simulink model "EulerKinematicalEquations"  (R2021a)
settings: Solver=FixedStepAuto  StartTime=0.0  StopTime=100  FixedStep=.05  RelTol=1e-3
values from neighbouring files (symbols this model uses):
  Cbv0 = Cb2*C21*C1v    [InitializeModel.m]
  phi0 = 0    [InitializeModel.m]
  psi0 = 0    [InitializeModel.m]
  theta0 = 0.0059    [InitializeModel.m]
settings Model: Creator=Christopher  LastModifiedBy=chris
settings SolverCC: AlgebraicLoopSolver=TrustRegion
settings DataIOCC: ReturnWorkspaceOutputs=off
settings DebuggingCC: SFMachineParentedDataDiag=warning  ArithmeticOperatorsInVariantConditions=warning
settings SFSimCC: CustomCodeUndefinedFunction=UseInterfaceOnly

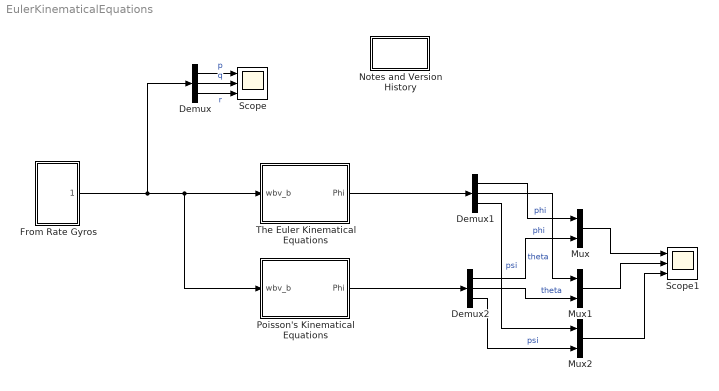
== system EulerKinematicalEquations ==
  Demux : Demux  Outputs=3
  Demux1 : Demux  Outputs=3
  Demux2 : Demux  Outputs=3
  From Rate Gyros : Subsystem
  Mux : Mux  Inputs=2
  Mux1 : Mux  Inputs=2
  Mux2 : Mux  Inputs=2
  Notes and Version History : Subsystem
  Poisson's Kinematical Equations : Subsystem
  Scope : Scope  NumInputPorts=3
  Scope1 : Scope  NumInputPorts=3
  The Euler Kinematical Equations : Subsystem
  wires:
  From Rate Gyros/1(wbv_b) -> Poisson's Kinematical Equations/1(wbv_b), The Euler Kinematical Equations/1(wbv_b), Demux/1
  Demux/1 -> Scope/1  "p"
  Demux/2 -> Scope/2  "q"
  Demux/3 -> Scope/3  "r"
  Demux1/3 -> Mux2/1  "psi"
  Demux1/2 -> Mux1/1  "theta"
  Demux1/1 -> Mux/1  "phi"
  The Euler Kinematical Equations/1(Phi) -> Demux1/1
  Poisson's Kinematical Equations/1(Phi) -> Demux2/1
  Demux2/1 -> Mux/2  "phi"
  Mux/1 -> Scope1/1
  Demux2/2 -> Mux1/2  "theta"
  Mux1/1 -> Scope1/2
  Demux2/3 -> Mux2/2  "psi"
  Mux2/1 -> Scope1/3

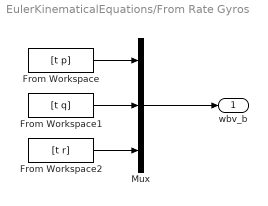
== system EulerKinematicalEquations/From Rate Gyros ==
  From Workspace : FromWorkspace  VariableName=[t p]
  From Workspace1 : FromWorkspace  VariableName=[t q]
  From Workspace2 : FromWorkspace  VariableName=[t r]
  Mux : Mux  Inputs=3
  wbv_b : Outport  VectorParamsAs1DForOutWhenUnconnected=off
  wires:
  From Workspace/1 -> Mux/1
  From Workspace1/1 -> Mux/2
  Mux/1 -> wbv_b/1
  From Workspace2/1 -> Mux/3

== system EulerKinematicalEquations/Notes and Version History ==
  note: Illustrate Euler Kinematical Equations and Poisson's Kinematical Equations
      |
      | Christopher Lum
      | lum@uw.edu
      |
      | Version History
      | 03/30/20: Created
      | 12/23/23: Moved to YouTube GitHub

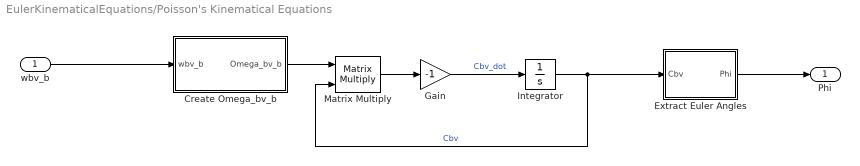
== system EulerKinematicalEquations/Poisson's Kinematical Equations ==
  wbv_b : Inport
  Create Omega_bv_b : MATLAB Function  TreatAsAtomicUnit=on
  Extract Euler Angles : MATLAB Function  TreatAsAtomicUnit=on
  Gain : Gain  Gain=-1
  Integrator : Integrator  InitialCondition=Cbv0
  Matrix Multiply : Product  Multiplication=Matrix(*)
  Phi : Outport  VectorParamsAs1DForOutWhenUnconnected=off
  wires:
  Create Omega_bv_b/1(Omega_bv_b) -> Matrix Multiply/1
  wbv_b/1 -> Create Omega_bv_b/1(wbv_b)
  Matrix Multiply/1 -> Gain/1
  Integrator/1 -> Matrix Multiply/2, Extract Euler Angles/1(Cbv)  "Cbv"
  Extract Euler Angles/1(Phi) -> Phi/1
  Gain/1 -> Integrator/1  "Cbv_dot"

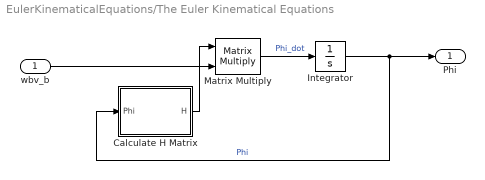
== system EulerKinematicalEquations/The Euler Kinematical Equations ==
  wbv_b : Inport
  Calculate H Matrix : MATLAB Function  TreatAsAtomicUnit=on
  Integrator : Integrator  InitialCondition=[phi0;theta0;psi0]
  Matrix Multiply : Product  Multiplication=Matrix(*)
  Phi : Outport  VectorParamsAs1DForOutWhenUnconnected=off
  wires:
  Integrator/1 -> Phi/1, Calculate H Matrix/1(Phi)  "Phi"
  Matrix Multiply/1 -> Integrator/1  "Phi_dot"
  wbv_b/1 -> Matrix Multiply/2
  Calculate H Matrix/1(H) -> Matrix Multiply/1

== matlab function EulerKinematicalEquations/The Euler Kinematical Equations/Calculate H Matrix ==
  data: Phi input; H output
function H = fcn(Phi)

%Unpack Phi
phi     = Phi(1);
theta   = Phi(2);
psi     = Phi(3);

%Input the H matrix
H = [1 tan(theta)*sin(phi) tan(theta)*cos(phi);
    0 cos(phi) -sin(phi);
    0 sin(phi)/cos(theta) cos(phi)/cos(theta)];

== matlab function EulerKinematicalEquations/Poisson's Kinematical Equations/Extract Euler Angles ==
  data: Cbv input; Phi output
function Phi = fcn(Cbv)

c11 = Cbv(1,1);
c13 = Cbv(1,3);
c12 = Cbv(1,2);
c23 = Cbv(2,3);
c33 = Cbv(3,3);

phi     = atan2(c23,c33);
theta   = -asin(c13);
psi2    = atan2(c12,c11);   %avoid problem with function called psi

Phi = [phi;theta;psi2];

== matlab function EulerKinematicalEquations/Poisson's Kinematical Equations/Create Omega_bv_b ==
  data: wbv_b input; Omega_bv_b output
function Omega_bv_b = fcn(wbv_b)

p = wbv_b(1);
q = wbv_b(2);
r = wbv_b(3);

Omega_bv_b = [0 -r q;
    r 0 -p;
    -q p 0];
